simulink model "Solar_Farm_simulink"  (R2023a)
settings: Solver=FixedStepDiscrete  StartTime=0.0  StopTime=2.5  RelTol=1e-3
PreLoadFcn:
  | Ts_Power=1e-6;
  | Ts_Control=100e-6;
InitFcn:
  | Ts_Power=1e-6;
  | Ts_Control=100e-6;
undefined symbols (not defined in the file): D1, Delta, DiscIntNeverNeededParam
libraries: spsSeriesRLCBranchLib x5, spsMeanLib x3, spsThreePhaseTransformerTwoWindingsLib x2, spsDistributedParametersLineLib x2, spsThreePhaseParallelRLCLoadLib x2, spsFourierLib x2, slpidlib x2, spsabctodq0Lib x2, spsVoltageMeasurementLib x2, spsThreePhaseSeriesRLCLoadLib x1, spsThreeLevelBridgeLib x1, spsThreePhaseSourceLib x1
(part 1 of 2)
settings Model: SimulationMode=accelerator  Creator=The MathWorks, Inc.
settings SolverCC: AlgebraicLoopSolver=TrustRegion
settings DataIOCC: LimitDataPoints=on  SaveFormat=Array  SignalLogging=off  DSMLogging=off  ReturnWorkspaceOutputs=off
settings OptimizationCC: ExpressionDepthLimit=2147483647  EfficientMapNaN2IntZero=off  LifeSpan=inf
settings DebuggingCC: UnderspecifiedInitializationDetection=Classic  MergeDetectMultiDrivingBlocksExec=none  SolverPrmCheckMsg=warning  FcnCallInpInsideContextMsg=warning  UnconnectedInputMsg=warning  UnconnectedOutputMsg=warning  UnconnectedLineMsg=warning  StateNameClashWarn=warning  SFUnexpectedBacktrackingDiag=warning  SFNoUnconditionalDefaultTransitionDiag=warning  SFExecutionAtInitializationDiag=none  ArithmeticOperatorsInVariantConditions=warning
settings HardwareCC: ProdBitPerPointer=32  ProdBitPerSizeT=32  ProdBitPerPtrDiffT=32  ProdLargestAtomicFloat=None  ProdIntDivRoundTo=Undefined  ProdEndianess=Unspecified  ProdWordSize=32  ProdHWDeviceType=32-bit Generic  TargetBitPerLong=64  TargetBitPerPointer=64  TargetBitPerSizeT=64  TargetBitPerPtrDiffT=64  TargetLongLongMode=on  TargetIntDivRoundTo=Zero  TargetEndianess=LittleEndian  TargetWordSize=64  TargetHWDeviceType=MATLAB Host  ProdEqTarget=off
settings ModelReferenceCC: EnableRefExpFcnMdlSchedulingChecks=on  PropagateSignalLabelsOutOfModel=off
settings SFSimCC: SimUseLocalCustomCode=off  CustomCodeUndefinedFunction=UseInterfaceOnly
settings CodeAppCC: MaxIdLength=128
settings GRTTargetCC: TargetLangStandard=C89/C90 (ANSI)  CombineOutputUpdateFcns=off  GRTInterface=on
settings ConfigComp: CovMetricSettings=dw  CovSaveCumulativeToWorkspaceVar=on  CovSaveSingleToWorkspaceVar=on  CovExternalEMLEnable=off  CovSFcnEnable=off
settings SimscapeCC: SimscapeNormalizeSystem=off

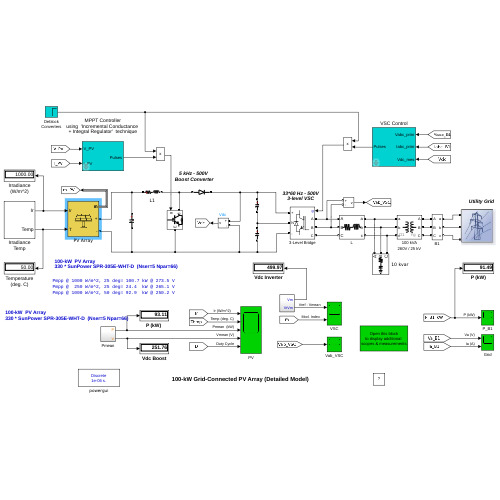
[thumbnail: Simulink's stored preview of the top-level diagram]
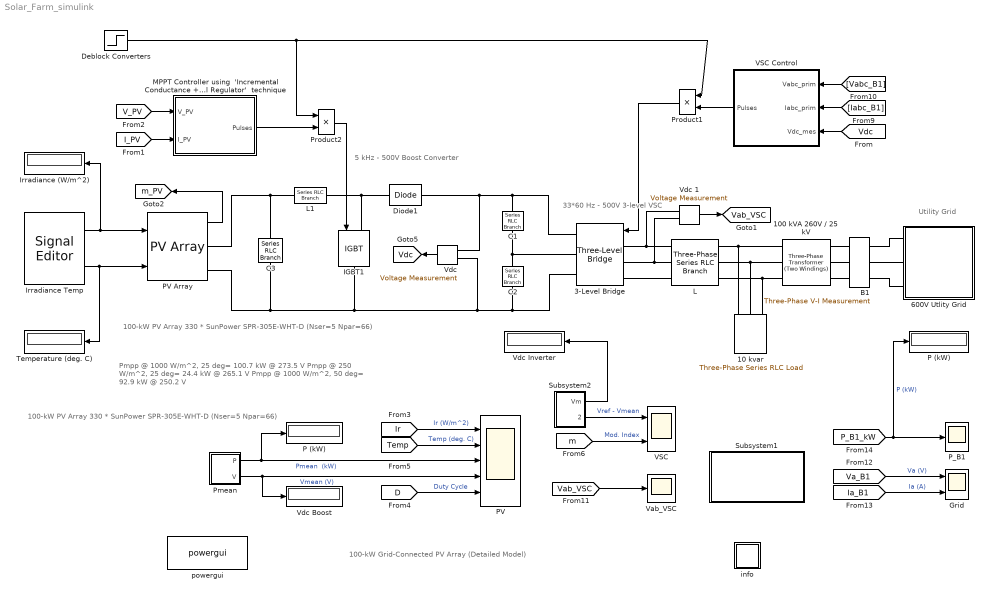
== system Solar_Farm_simulink ==
  note: 5 kHz - 500V
      | Boost Converter
  note: 33*60 Hz - 500V
      | 3-level VSC
  note: 100-kW Grid-Connected PV Array (Detailed Model)
  note: Utility Grid
  note: Pmpp @ 1000 W/m^2, 25 deg= 100.7 kW @ 273.5 V
      | Pmpp @  250 W/m^2, 25 deg= 24.4  kW @ 265.1 V
      | Pmpp @ 1000 W/m^2, 50 deg= 92.9  kW @ 250.2 V
  note: 100-kW  PV Array
      | 330 * SunPower SPR-305E-WHT-D  (Nser=5 Npar=66)
  note: 100-kW  PV Array
      | 330 * SunPower SPR-305E-WHT-D  (Nser=5 Npar=66)
  10 kvar : spsThreePhaseSeriesRLCLoadLib/Three-Phase Series RLC Load  LConnTagsString=A|B|C  Configuration=Y (grounded)  NominalVoltage=240  Vabc=[1e3 1e3 1e3]  Vabcp=[1e3 1e3 1e3]  NominalFrequency=60  UnbalancedPower=off  ActivePower=10e3/100  InductivePower=0  CapacitivePower=10e3  Pabc=[10e3 9e3 11e3]  QLabc=[100 90 110]  QCabc=[100 90 110]  Pabcp=[10e3 9e3 11e3]  QLabcp=[100 90 110]  QCabcp=[100 90 110]  Measurements=None  LoadType=constant Z
  100 kVA 260V / 25 kV : spsThreePhaseTransformerTwoWindingsLib/Three-Phase Transformer (Two Windings)  Winding1Connection=Yg  Winding2Connection=Delta (D1)  CoreType=Three single-phase transformers  SetSaturation=off  Hysteresis=off  DataFile='hysteresis'  SetInitialFlux=off  Measurements=None  UNITS=pu  NominalPower=[100e3 , 60 ]  Winding1=[ 25e3 , 0.001 , 0.03 ]  Winding2=[ 260 , 0.001 , 0.03 ]  Rm=500  Lm=500  L0=0.5  Saturation=[ 0,0 ; 0.0024,1.2 ; 1.0,1.52 ]  InitialFluxes=[ 0.8 , -0.8 , 0.7 ]  BreakLoop=off  DiscreteSolver=Trapezoidal iterative  DataType=off  TransfoNumber=0
  3-Level Bridge : spsThreeLevelBridgeLib/Three-Level Bridge  Arms=3  SnubberResistance=1e6  SbubberCapacitance=inf  Device=IGBT / Diodes  Ron=0.2e-3  ForwardVoltages="[  0  0 ]"  Measurements=None
      settings: AttributesFormatString=\n
  600V Utlity Grid : Subsystem
      mask Display: image('grid.jpg')
  B1 : spsThreePhaseVIMeasurementLib/Three-Phase V-I Measurement  VoltageMeasurement=phase-to-ground  SetLabelV=on  LabelV=Vabc_B1  Vpu=off  VpuLL=off  CurrentMeasurement=yes  SetLabelI=on  LabelI=Iabc_B1  Ipu=off  Pbase=100e6  Vbase=500e3  OutputType=Magnitude  PhasorSimulation=off  PSBequivalent=0
  C1 : spsSeriesRLCBranchLib/Series RLC Branch  LConnTagsString=__new0  RConnTagsString=__new0  BranchType=C  Resistance=1.0  Inductance=1.0  SetiL0=off  InitialCurrent=0  Capacitance=12000e-06  Setx0=off  InitialVoltage=0  Measurements=None
  C2 : spsSeriesRLCBranchLib/Series RLC Branch  LConnTagsString=__new0  RConnTagsString=__new0  BranchType=C  Resistance=1.0  Inductance=1.0  SetiL0=off  InitialCurrent=0  Capacitance=12000e-06  Setx0=off  InitialVoltage=0  Measurements=None
  C3 : spsSeriesRLCBranchLib/Series RLC Branch  LConnTagsString=__new0  RConnTagsString=__new0  BranchType=C  Resistance=1.0  Inductance=1.0  SetiL0=off  InitialCurrent=0  Capacitance=100e-6  Setx0=off  InitialVoltage=0  Measurements=Branch voltage
  Deblock Converters : Step  Time=0.05  SampleTime=0
  Diode1 : spsDiodeLib/Diode  Ron=1e-4  Lon=0  Vf=0  IC=0  UseSnubber=off  Rs=inf  Cs=inf  Measurements=off
  Grid : Scope  NumInputPorts=2
  IGBT1 : spsIGBTLib/IGBT  Ron=0.001  Lon=0  Vf=0  Tf=0  Tt=0  IC=0  Rs=1e5  Cs=inf  Measurements=off
  Irradiance (W/m^2) : Display
      settings: Format=bank  Decimation=1000
  Irradiance Temp : SignalEditorBlockLib/Signal Editor  FileName=dpower_PVarray_grid_det.mat  ActiveScenario=Ramp_up_down_Irradiance  ActiveSignal=Temp  IsBus=off  OutputBusObjectStr=Bus: BusObject  SampleTime=0  OutputAfterFinalValue=Extrapolation  Unit=inherit  PreserveSignalName=on  ApplySigPropsToAllScenarios=on
  L : spsThreePhaseSeriesRLCBranchLib/Three-Phase Series RLC Branch  LConnTagsString=A|B|C  RConnTagsString=A|B|C  BranchType=RL  Resistance=500e-6*377/50/2  Inductance=500e-6/2  Capacitance=inf  Measurements=None
  L1 : spsSeriesRLCBranchLib/Series RLC Branch  LConnTagsString=__new0  RConnTagsString=__new0  BranchType=RL  Resistance=0.005  Inductance=5e-3  SetiL0=off  InitialCurrent=0  Capacitance=1e-6  Setx0=off  InitialVoltage=0  Measurements=None
  "MPPT Controller using  'Incremental Conductance + Integral Regulator'  technique " : Subsystem  mask(Boost Control - MPPT){fc=5000, T_MPPT=200e-6, Dinit=0.5}
      mask prompts: fc "PWM switching frequency (Hz)"; T_MPPT "Time window used by MPPT control (s)"; Dinit "Initial value of duty cycle"
  P (kW) : Display
      settings: Format=bank  Decimation=2000
  "P (kW) " : Display
      settings: Format=bank  Decimation=2000
  PV : Scope  NumInputPorts=5
  PV Array : spsPVArrayLib/PV Array  Npar=66  Nser=5  PlotType=array @ 1000 W/m2 & specified temperatures  S_vec="[ 1000  250 ]"  Temp_C_vec="[0 25  50  ]"  ModuleName=SunPower SPR-305E-WHT-D  PlotWhenSelected=off  Pm=305.226  Ncell=96  Voc=64.2  Isc=5.96  Vm=54.7  Im=5.58  beta_Voc_pc=-0.2727  alpha_Isc_pc=0.061745  beta_Voc=-0.17507  alpha_Isc=0.00368  IL=5.9657  I0=6.3076e-12  nI=0.94489  Rsh=393.2054  Rs=0.37428  RobustModel=off  RobustCellTemperature=25  BAL=on  Tc=1e-6  Tfilter=5e-5
  P_B1 : Scope
  Pmean : Subsystem
  Product1 : Product  RndMeth=Zero
  Product2 : Product  RndMeth=Zero
  Subsystem1 : Subsystem
      mask Display: disp('Open this block\nto display additional \nscopes & measurements')
  Subsystem2 : Subsystem
  Temperature (deg. C) : Display
      settings: Format=bank  Decimation=1000
  VSC : Scope  NumInputPorts=2
  VSC Control : Subsystem  mask(VSC Main Controller){nom=[ 100e3  60 ], Vnom=[ 25e3 260 ], Vnom_dc=500, RLxfo=[0.002  0.06 ], RLchoke=[2e-3  250e-6  ], K_VDCreg=[7  800], K_Ireg=[0.3 20], Ts=Ts_Control}
      mask prompts: nom "Nominal power and frequency [ Pnom(VA)  Fnom(Hz) ]:"; Vnom "Nominal primary and secondary voltages (Vrms LL) [ Vnom_prim   Vnom_sec ]:"; Vnom_dc "Nominal DC bus voltage (V):"; RLxfo "Total transformer leakage impedance (pu/Pnom) [ Rxfo  Lxf ]"; RLchoke "Choke impedance [ R(ohm) L(H) ]"; K_VDCreg "VDC regultator gains [ Kp  Ki ]:"; K_Ireg "Current regulator gains [ Kp  Ki ]:"; Ts "Sample time"
      mask init:
      | Pnom=nom(1);
      | Fnom=nom(2);
      | Vnom_prim=Vnom(1);
      | Vnom_sec=Vnom(2);
      | Zbase=Vnom_sec^2/Pnom;
      | Rtot_pu=RLxfo(1) + RLchoke(1)/Zbase;
      | Ltot_pu=RLxfo(2) + RLchoke(2)/(Zbase/(2*pi*Fnom));
      | Kp_VDCreg=K_VDCreg(1);
      | Ki_VDCreg=K_VDCreg(2);
      | Kp_Ireg=K_Ireg(1);
      | Ki_Ireg=K_Ireg(2);
      | Vdc_ref=Vnom_dc;
      | % Used to determine initial value of Boost Control (MPPT)
      | assignin('base','Vdc_ref_Inv',Vdc_ref);
  Vab_VSC : Scope
  "Vdc " : spsVoltageMeasurementLib/Voltage Measurement  Tag=PoWeRsYsTeMmEaSuReMeNt  PhasorSimulation=off  OutputType=Magnitude  PSBequivalent=0
  Vdc 1 : spsVoltageMeasurementLib/Voltage Measurement  Tag=PoWeRsYsTeMmEaSuReMeNt  PhasorSimulation=off  OutputType=Magnitude  PSBequivalent=0
  Vdc Boost : Display
      settings: Format=bank  Decimation=2000
  Vdc Inverter : Display
      settings: Format=bank  Decimation=2000
  info : Subsystem
      settings: OpenFcn=showdemo(bdroot(gcb))
      mask Display: disp('?')
  powergui : spspowerguiLib/powergui  Priority=1  SimulationMode=Discrete  SampleTime=Ts_Power  frequency=60  Iterations=50  frequencyindice=0  Pbase=100e6  ErrMax=1e-4  UnitsV=kV  UnitsW=MW  buscounter=0  FunctionMessages=off  echomessages=off  EnableUseOfTLC=off  CurrentSourceSwitches=off  DisableSnubberDevices=off  DisableRonSwitches=off  DisableVfSwitches=off  DisplayEquations=off  AutomaticDiscreteSolvers=off  SolverType=Tustin/Backward Euler (TBE)  Interpol=off  ExternalGateDelay=off  methode=off  Ts=0  x0status=blocks  SPID=off  SwTol=0  HookPort=off  NonlinearTolerance=1e-8  nMaxIteration=10  ContinueOnMaxIteration=off  RestoreLinks=warning  ResistiveCurrentMeasurement=off  Frange=[0:2:500]  Ylog=off  Xlog=on  ShowGrid=off  save=off  variable=ZData  structure=0  ZoomFFT=on  StartTime=0.0  cycles=1  DisplayStyle=1  fundamental=60  FreqAxis=off  MaxFrequency=1000  frequencyindicesteady=1  RmsSteady=1  display=off
  tag scope: Vab_VSC=global, Vdc=global, m_PV=global
  wires:
  "Vdc "/1 -> [Vdc]
  Product2/1 -> IGBT1/1
  "MPPT Controller using  'Incremental Conductance + Integral Regulator'  technique "/1(Pulses) -> Product2/2
  Deblock Converters/1 -> Product1/1, Product2/1
  [Vabc_B1] -> VSC Control/1(Vabc_prim)
  [Iabc_B1] -> VSC Control/2(Iabc_prim)
  [Vdc] -> VSC Control/3(Vdc_mes)
  VSC Control/1(Pulses) -> Product1/2
  Product1/1 -> 3-Level Bridge/1
  [I_PV] -> "MPPT Controller using  'Incremental Conductance + Integral Regulator'  technique "/2(I_PV)
  [V_PV] -> "MPPT Controller using  'Incremental Conductance + Integral Regulator'  technique "/1(V_PV)
  Pmean/1(P) -> "P (kW) "/1, PV/3  "Pmean  (kW)"
  [m] -> VSC/2  "Mod. Index"
  Vdc 1/1 -> [Vab_VSC]
  [Vab_VSC] -> Vab_VSC/1
  [Ia_B1] -> Grid/2  "Ia (A)"
  [Va_B1] -> Grid/1  "Va (V)"
  [P_B1_kW] -> P_B1/1, P (kW)/1  "P (kW)"
  Pmean/2(V) -> Vdc Boost/1, PV/4  "Vmean (V)"
  Subsystem2/2(VrVm) -> VSC/1  "Vref - Vmean"
  Subsystem2/1(Vm) -> Vdc Inverter/1
  PV Array/1 -> [m_PV]
  Irradiance Temp/1 -> PV Array/1, Irradiance (W/m^2)/1
  Irradiance Temp/2 -> PV Array/2, Temperature (deg. C)/1
  [D] -> PV/5  "Duty Cycle"
  [Temp] -> PV/2  "Temp (deg. C)"
  [Ir] -> PV/1  "Ir (W/m^2)"
  connections:
  3-Level Bridge/RConn1 -- Diode1/RConn1 -- "Vdc "/LConn1 -- C1/LConn1
  L1/RConn1 -- Diode1/LConn1 -- IGBT1/LConn1
  3-Level Bridge/RConn3 -- C2/RConn1 -- "Vdc "/LConn2 -- IGBT1/RConn1 -- PV Array/RConn2 -- C3/RConn1
  3-Level Bridge/LConn1 -- L/LConn1 -- Vdc 1/LConn1
  3-Level Bridge/LConn2 -- L/LConn2 -- Vdc 1/LConn2
  3-Level Bridge/LConn3 -- L/LConn3
  L/RConn1 -- 100 kVA 260V / 25 kV/RConn1 -- 10 kvar/LConn1
  L/RConn2 -- 100 kVA 260V / 25 kV/RConn2 -- 10 kvar/LConn2
  L/RConn3 -- 100 kVA 260V / 25 kV/RConn3 -- 10 kvar/LConn3
  B1/LConn1 -- 100 kVA 260V / 25 kV/LConn1
  B1/LConn2 -- 100 kVA 260V / 25 kV/LConn2
  B1/LConn3 -- 100 kVA 260V / 25 kV/LConn3
  C2/LConn1 -- C1/RConn1 -- 3-Level Bridge/RConn2
  C3/LConn1 -- PV Array/RConn1 -- L1/LConn1
  B1/RConn2 -- 600V Utlity Grid/LConn2
  B1/RConn1 -- 600V Utlity Grid/LConn1
  B1/RConn3 -- 600V Utlity Grid/LConn3

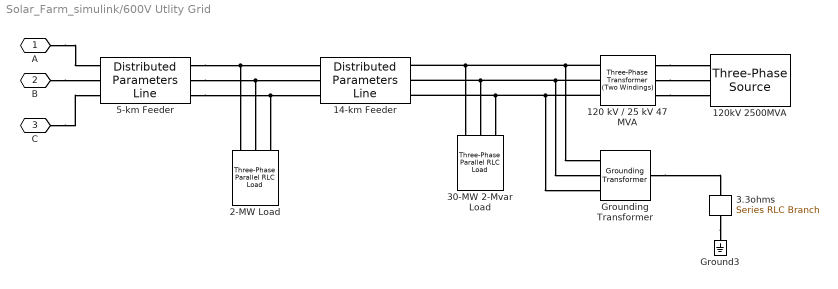
== system Solar_Farm_simulink/600V Utlity Grid ==
  120 kV / 25 kV 47 MVA : spsThreePhaseTransformerTwoWindingsLib/Three-Phase Transformer (Two Windings)  Winding1Connection=Yg  Winding2Connection=Delta (D1)  CoreType=Three single-phase transformers  SetSaturation=off  Hysteresis=off  DataFile='basic_model'  SetInitialFlux=off  Measurements=None  UNITS=pu  NominalPower=[47e6 60 ]  Winding1="[ 120e3  0.08/30   0.08 ]"  Winding2="[ 25e3  0.08/30  0.08]"  Rm=500  Lm=500  L0=0.5  Saturation="[ 0,0  ;  0.005,1.2  ;  1.0,1.4 ]"  InitialFluxes=[ 0.8 , -0.8 , 0.7 ]  BreakLoop=off  DiscreteSolver=Trapezoidal iterative  DataType=off  TransfoNumber=0
  120kV 2500MVA : spsThreePhaseSourceLib/Three-Phase Source  InternalConnection=Yg  VoltagePhases=off  Voltage=120e3  PhaseAngle=0  Voltage_phases=[25e3 25e3 25e3]/sqrt(3)  PhaseAngles_phases=[0 -120 +120]  Frequency=60  NonIdealSource=on  SpecifyImpedance=on  Resistance=0.8929  Inductance=16.58e-3  ShortCircuitLevel=2500e6  BaseVoltage=120e3  XRratio=7  BusType=swing  Pref=0  Qref=0  Prefabc=[10e3, 10e3, 10e3]  Qrefabc=[0, 0, 0]  Qmin=-inf  Qmax=inf
  14-km Feeder : spsDistributedParametersLineLib/Distributed Parameters Line  Phases=3  Length=14  Frequency=60  Resistance=[0.1153 0.413]  Inductance=[1.05e-3 3.32e-3]  Capacitance=[11.33e-009 5.01e-009]  x1=[-5.8e-05 2.50217396067509e-09 0 0;-5.7e-05 2.50196188940633e-09 0 0;-5.6e-05 2.50174946255299e-09 0 0;-5.5e-05 2.50153668014525e-09 0 0;-5.4e-05 2.50132354221337e-09 0 0;-5.3e-05 2.50111004878763e-09 0 0;-5.2e-05 2.50089619989837e-09 0 0;-5.1e-05 2.50068199557598e-09 0 0;-5e-05 2.50046743585092e-09 0 0;-4.9e-05 2.50025252075366e-09 -3790.73535189975 -24061.4134200279;-4.8e-05 2.50003725031477e-09 -3781.66414358436 -24062.8407837223;-4.7e-05 2.49982162456482e-09 -3772.59239781015 -24064.2647275504;-4.6e-05 2.49960564353448e-09 -3763.52011586643 -24065.6852513098;-4.5e-05 2.49938930725442e-09 -3754.44729904257 -24067.1023547986;-4.4e-05 2.49917261575541e-09 -3745.37394862801 -24068.5160378155;-4.3e-05 2.49895556906823e-09 -3736.30006591229 -24069.9263001594;-4.2e-05 2.49873816722373e-09 -3727.225652185 -24071.33314163;-4.1e-05 2.49852041025281e-09 -3718.15070873583 -24072.7365620274;-4e-05 2.49830229818642e-09 -3709.07523685452 -24074.136561152;-3.9e-05 2.49808383105556e-09 -3699.99923783089 -24075.5331388049;-3.8e-05 2.49786500889127e-09 -3690.92271295487 -24076.9262947876;-3.7e-05 2.49764583172466e-09 -3681.8456635164 -24078.3160289022;-3.6e-05 2.49742629958688e-09 -3672.76809080556 -24079.702340951;-3.5e-05 2.49720641250912e-09 -3663.68999611247 -24081.0852307371;-3.4e-05 2.49698617052264e-09 -3654.61138072732 -24082.464698064;-3.3e-05 2.49676557365874e-09 -3645.53224594039 -24083.8407427356;-3.2e-05 2.49654462194876e-09 -3636.45259304202 -24085.2133645562;-3.1e-05 2.49632331542412e-09 -3627.37242332264 -24086.582563331;-3e-05 2.49610165411627e-09 -3618.29173807275 -24087.9483388651;-2.9e-05 2.4958796380567e-09 -3609.2105385829 -24089.3106909646;-2.8e-05 2.49565726727697e-09 -3600.12882614375 -24090.6696194359;-2.7e-05 2.49543454180869e-09 -3591.046602046 -24092.0251240857;-2.6e-05 2.4952114616835e-09 -3581.96386758044 -24093.3772047214;-2.5e-05 2.49498802693312e-09 -3572.88062403793 -24094.7258611509;-2.4e-05 2.4947642375893e-09 -3563.7968727094 -24096.0710931825;-2.3e-05 2.49454009368384e-09 -3554.71261488586 -24097.4129006251;-2.2e-05 2.49431559524861e-09 -3545.62785185838 -24098.7512832878;-2.1e-05 2.4940907423155e-09 -3536.54258491811 -24100.0862409806;-2e-05 2.49386553491647e-09 -3527.45681535627 -24101.4177735136;-1.9e-05 2.49363997308353e-09 -3518.37054446415 -24102.7458806977;-1.8e-05 2.49341405684874e-09 -3509.2837735331 -24104.070562344;-1.7e-05 2.49318778624421e-09 -3500.19650385457 -24105.3918182643;-1.6e-05 2.49296116130209e-09 -3491.10873672006 -24106.7096482709;-1.5e-05 2.49273418205459e-09 -3482.02047342113 -24108.0240521764;-1.4e-05 2.49250684853397e-09 -3472.93171524945 -24109.3350297941;-1.3e-05 2.49227916077254e-09 -3463.84246349671 -24110.6425809375;-1.2e-05 2.49205111880266e-09 -3454.75271945471 -24111.946705421;-1.1e-05 2.49182272265674e-09 -3445.6624844153 -24113.247403059;-1e-05 2.49159397236724e-09 -3436.57175967041 -24114.5446736669;-9e-06 2.49136486796667e-09 -3427.48054651203 -24115.8385170602;-8e-06 2.49113540948759e-09 -3418.38884623222 -24117.1289330549;-7e-06 2.49090559696261e-09 -3409.29666012313 -24118.4159214678;-6e-06 2.49067543042439e-09 -3400.20398947694 -24119.699482116;-5e-06 2.49044490990565e-09 -3391.11083558594 -24120.9796148169;-4e-06 2.49021403543915e-09 -3382.01719974246 -24122.2563193887;-3e-06 2.48998280705769e-09 -3372.92308323891 -24123.5295956499;-2e-06 2.48975122479415e-09 -3363.82848736777 -24124.7994434195;-1e-06 2.48951928868143e-09 -3354.73341342159 -24126.0658625171]  x2=[-5.8e-05 2.62043607139288e-09 0 0;-5.7e-05 2.62017695324581e-09 0 0;-5.6e-05 2.61991746271315e-09 0 0;-5.5e-05 2.61965759983179e-09 0 0;-5.4e-05 2.61939736463867e-09 0 0;-5.3e-05 2.61913675717076e-09 0 0;-5.2e-05 2.61887577746511e-09 0 0;-5.1e-05 2.6186144255588e-09 0 0;-5e-05 2.61835270148898e-09 0 0;-4.9e-05 2.61809060529286e-09 -3379.39242591326 -24244.0512732181;-4.8e-05 2.61782813700767e-09 -3370.25239398146 -24245.323551308;-4.7e-05 2.61756529667072e-09 -3361.11188306163 -24246.5923835967;-4.6e-05 2.61730208431936e-09 -3351.97089445284 -24247.8577699039;-4.5e-05 2.61703849999101e-09 -3342.82942945423 -24249.1197100497;-4.4e-05 2.61677454372312e-09 -3333.68748936501 -24250.3782038548;-4.3e-05 2.61651021555321e-09 -3324.54507548445 -24251.6332511404;-4.2e-05 2.61624551551885e-09 -3315.4021891119 -24252.884851728;-4.1e-05 2.61598044365765e-09 -3306.25883154675 -24254.1330054398;-4e-05 2.61571500000729e-09 -3297.11500408849 -24255.3777120984;-3.9e-05 2.6154491846055e-09 -3287.97070803665 -24256.6189715269;-3.8e-05 2.61518299749005e-09 -3278.82594469085 -24257.8567835489;-3.7e-05 2.61491643869877e-09 -3269.68071535076 -24259.0911479884;-3.6e-05 2.61464950826954e-09 -3260.53502131612 -24260.3220646701;-3.5e-05 2.61438220624031e-09 -3251.38886388674 -24261.5495334189;-3.4e-05 2.61411453264907e-09 -3242.24224436249 -24262.7735540605;-3.3e-05 2.61384648753385e-09 -3233.09516404331 -24263.9941264209;-3.2e-05 2.61357807093275e-09 -3223.9476242292 -24265.2112503265;-3.1e-05 2.61330928288392e-09 -3214.79962622023 -24266.4249256045;-3e-05 2.61304012342556e-09 -3205.65117131655 -24267.6351520823;-2.9e-05 2.61277059259592e-09 -3196.50226081834 -24268.841929588;-2.8e-05 2.61250069043331e-09 -3187.35289602587 -24270.04525795;-2.7e-05 2.61223041697609e-09 -3178.20307823947 -24271.2451369973;-2.6e-05 2.61195977226267e-09 -3169.05280875954 -24272.4415665594;-2.5e-05 2.61168875633152e-09 -3159.90208888652 -24273.6345464662;-2.4e-05 2.61141736922115e-09 -3150.75091992095 -24274.8240765482;-2.3e-05 2.61114561097013e-09 -3141.5993031634 -24276.0101566363;-2.2e-05 2.61087348161709e-09 -3132.44723991454 -24277.192786562;-2.1e-05 2.6106009812007e-09 -3123.29473147505 -24278.3719661572;-2e-05 2.61032810975968e-09 -3114.14177914574 -24279.5476952542;-1.9e-05 2.61005486733283e-09 -3104.98838422742 -24280.7199736861;-1.8e-05 2.60978125395898e-09 -3095.83454802101 -24281.8888012861;-1.7e-05 2.609507269677e-09 -3086.68027182747 -24283.0541778883;-1.6e-05 2.60923291452585e-09 -3077.52555694782 -24284.2161033268;-1.5e-05 2.60895818854451e-09 -3068.37040468316 -24285.3745774367;-1.4e-05 2.60868309177202e-09 -3059.21481633464 -24286.5296000533;-1.3e-05 2.60840762424749e-09 -3050.05879320346 -24287.6811710123;-1.2e-05 2.60813178601007e-09 -3040.9023365909 -24288.8292901503;-1.1e-05 2.60785557709895e-09 -3031.74544779831 -24289.9739573039;-1e-05 2.6075789975534e-09 -3022.58812812708 -24291.1151723104;-9e-06 2.60730204741271e-09 -3013.43037887866 -24292.2529350078;-8e-06 2.60702472671626e-09 -3004.27220135458 -24293.3872452343;-7e-06 2.60674703550346e-09 -2995.11359685643 -24294.5181028287;-6e-06 2.60646897381376e-09 -2985.95456668583 -24295.6455076302;-5e-06 2.6061905416867e-09 -2976.7951121445 -24296.7694594787;-4e-06 2.60591173916183e-09 -2967.63523453419 -24297.8899582144;-3e-06 2.6056325662788e-09 -2958.47493515674 -24299.007003678;-2e-06 2.60535302307726e-09 -2949.31421531402 -24300.1205957109;-1e-06 2.60507310959696e-09 -2940.15307630797 -24301.2307341546]  x3=[-5.8e-05 1.12841261134887e-11 0 0;-5.7e-05 1.12856673900563e-11 0 0;-5.6e-05 1.12872070626789e-11 0 0;-5.5e-05 1.12887451311376e-11 0 0;-5.4e-05 1.12902815952139e-11 0 0;-5.3e-05 1.12918164546894e-11 0 0;-5.2e-05 1.1293349709346e-11 0 0;-5.1e-05 1.12948813589657e-11 0 0;-5e-05 1.12964114033308e-11 0 0;-4.9e-05 1.1297939842224e-11 -23.5442847382639 -155.681477773843;-4.8e-05 1.1299466675428e-11 -23.4855925321452 -155.690342696964;-4.7e-05 1.13009919027257e-11 -23.4268969882001 -155.699185493015;-4.6e-05 1.13025155239005e-11 -23.3681981147704 -155.70800616074;-4.5e-05 1.13040375387357e-11 -23.3094959201986 -155.716804698884;-4.4e-05 1.13055579470151e-11 -23.2507904128276 -155.725581106197;-4.3e-05 1.13070767485226e-11 -23.1920816010008 -155.734335381433;-4.2e-05 1.13085939430424e-11 -23.133369493062 -155.743067523346;-4.1e-05 1.13101095303587e-11 -23.0746540973554 -155.751777530696;-4e-05 1.13116235102562e-11 -23.0159354222259 -155.760465402245;-3.9e-05 1.13131358825198e-11 -22.9572134760186 -155.769131136758;-3.8e-05 1.13146466469344e-11 -22.8984882670794 -155.777774733004;-3.7e-05 1.13161558032854e-11 -22.8397598037543 -155.786396189754;-3.6e-05 1.13176633513583e-11 -22.7810280943899 -155.794995505782;-3.5e-05 1.13191692909389e-11 -22.7222931473334 -155.803572679867;-3.4e-05 1.1320673621813e-11 -22.6635549709323 -155.81212771079;-3.3e-05 1.1322176343767e-11 -22.6048135735346 -155.820660597335;-3.2e-05 1.13236774565872e-11 -22.5460689634888 -155.829171338288;-3.1e-05 1.13251769600603e-11 -22.4873211491437 -155.837659932442;-3e-05 1.13266748539732e-11 -22.4285701388489 -155.846126378588;-2.9e-05 1.13281711381129e-11 -22.369815940954 -155.854570675524;-2.8e-05 1.1329665812267e-11 -22.3110585638093 -155.86299282205;-2.7e-05 1.13311588762228e-11 -22.2522980157657 -155.871392816968;-2.6e-05 1.13326503297683e-11 -22.1935343051743 -155.879770659086;-2.5e-05 1.13341401726914e-11 -22.1347674403867 -155.888126347211;-2.4e-05 1.13356284047804e-11 -22.0759974297549 -155.896459880157;-2.3e-05 1.13371150258238e-11 -22.0172242816317 -155.90477125674;-2.2e-05 1.13386000356103e-11 -21.9584480043698 -155.913060475777;-2.1e-05 1.13400834339289e-11 -21.8996686063228 -155.921327536092;-2e-05 1.13415652205688e-11 -21.8408860958444 -155.929572436509;-1.9e-05 1.13430453953193e-11 -21.7821004812891 -155.937795175856;-1.8e-05 1.13445239579701e-11 -21.7233117710114 -155.945995752964;-1.7e-05 1.1346000908311e-11 -21.6645199733668 -155.954174166669;-1.6e-05 1.13474762461321e-11 -21.6057250967106 -155.962330415807;-1.5e-05 1.13489499712238e-11 -21.5469271493991 -155.97046449922;-1.4e-05 1.13504220833766e-11 -21.4881261397888 -155.978576415752;-1.3e-05 1.13518925823813e-11 -21.4293220762364 -155.986666164249;-1.2e-05 1.13533614680289e-11 -21.3705149670995 -155.994733743563;-1.1e-05 1.13548287401107e-11 -21.3117048207358 -156.002779152545;-1e-05 1.1356294398418e-11 -21.2528916455036 -156.010802390054;-9e-06 1.13577584427427e-11 -21.1940754497615 -156.018803454949;-8e-06 1.13592208728765e-11 -21.1352562418686 -156.026782346091;-7e-06 1.13606816886118e-11 -21.0764340301845 -156.034739062349;-6e-06 1.13621408897408e-11 -21.017608823069 -156.04267360259;-5e-06 1.13635984760562e-11 -20.9587806288826 -156.050585965687;-4e-06 1.13650544473509e-11 -20.8999494559861 -156.058476150516;-3e-06 1.13665088034178e-11 -20.8411153127406 -156.066344155955;-2e-06 1.13679615440503e-11 -20.7822782075078 -156.074189980886;-1e-06 1.1369412669042e-11 -20.7234381486499 -156.082013624194]  x4=[-5.8e-05 -5.62786037485921e-12 0 0;-5.7e-05 -5.62923828223865e-12 0 0;-5.6e-05 -5.63061538957779e-12 0 0;-5.5e-05 -5.63199169668091e-12 0 0;-5.4e-05 -5.6333672033524e-12 0 0;-5.3e-05 -5.63474190939679e-12 0 0;-5.2e-05 -5.63611581461868e-12 0 0;-5.1e-05 -5.63748891882282e-12 0 0;-5e-05 -5.63886122181406e-12 0 0;-4.9e-05 -5.64023272339737e-12 -1.35581366009314 -2.15298522698133;-4.8e-05 -5.64160342337782e-12 -1.355001907458 -2.15349620368372;-4.7e-05 -5.6429733215606e-12 -1.35418996224687 -2.15400687432627;-4.6e-05 -5.64434241775103e-12 -1.35337782457515 -2.1545172388364;-4.5e-05 -5.64571071175452e-12 -1.35256549455825 -2.15502729714159;-4.4e-05 -5.64707820337661e-12 -1.35175297231164 -2.15553704916934;-4.3e-05 -5.64844489242295e-12 -1.35094025795078 -2.1560464948472;-4.2e-05 -5.6498107786993e-12 -1.35012735159118 -2.15655563410277;-4.1e-05 -5.65117586201154e-12 -1.34931425334838 -2.15706446686369;-4e-05 -5.65254014216565e-12 -1.34850096333792 -2.15757299305764;-3.9e-05 -5.65390361896775e-12 -1.34768748167541 -2.15808121261235;-3.8e-05 -5.65526629222406e-12 -1.34687380847645 -2.15858912545559;-3.7e-05 -5.6566281617409e-12 -1.34605994385669 -2.15909673151518;-3.6e-05 -5.65798922732473e-12 -1.34524588793178 -2.15960403071897;-3.5e-05 -5.65934948878211e-12 -1.34443164081744 -2.16011102299487;-3.4e-05 -5.66070894591971e-12 -1.34361720262937 -2.16061770827082;-3.3e-05 -5.66206759854433e-12 -1.34280257348334 -2.1611240864748;-3.2e-05 -5.66342544646287e-12 -1.34198775349511 -2.16163015753485;-3.1e-05 -5.66478248948234e-12 -1.3411727427805 -2.16213592137905;-3e-05 -5.6661387274099e-12 -1.34035754145533 -2.16264137793552;-2.9e-05 -5.66749416005277e-12 -1.33954214963546 -2.16314652713242;-2.8e-05 -5.66884878721833e-12 -1.33872656743677 -2.16365136889795;-2.7e-05 -5.67020260871405e-12 -1.33791079497519 -2.16415590316037;-2.6e-05 -5.67155562434753e-12 -1.33709483236664 -2.16466012984798;-2.5e-05 -5.67290783392646e-12 -1.3362786797271 -2.1651640488891;-2.4e-05 -5.67425923725868e-12 -1.33546233717256 -2.16566766021212;-2.3e-05 -5.67560983415212e-12 -1.33464580481903 -2.16617096374548;-2.2e-05 -5.67695962441482e-12 -1.33382908278257 -2.16667395941762;-2.1e-05 -5.67830860785495e-12 -1.33301217117925 -2.16717664715708;-2e-05 -5.67965678428079e-12 -1.33219507012518 -2.16767902689241;-1.9e-05 -5.68100415350074e-12 -1.33137777973647 -2.1681810985522;-1.8e-05 -5.68235071532331e-12 -1.33056030012929 -2.1686828620651;-1.7e-05 -5.6836964695571e-12 -1.32974263141982 -2.16918431735981;-1.6e-05 -5.68504141601088e-12 -1.32892477372426 -2.16968546436505;-1.5e-05 -5.68638555449348e-12 -1.32810672715886 -2.17018630300959;-1.4e-05 -5.68772888481389e-12 -1.32728849183987 -2.17068683322226;-1.3e-05 -5.68907140678117e-12 -1.32647006788359 -2.17118705493192;-1.2e-05 -5.69041312020452e-12 -1.32565145540633 -2.17168696806749;-1.1e-05 -5.69175402489327e-12 -1.32483265452443 -2.1721865725579;-1e-05 -5.69309412065684e-12 -1.32401366535426 -2.17268586833215;-9e-06 -5.69443340730476e-12 -1.32319448801223 -2.17318485531929;-8e-06 -5.6957718846467e-12 -1.32237512261475 -2.1736835334484;-7e-06 -5.69710955249243e-12 -1.32155556927827 -2.17418190264859;-6e-06 -5.69844641065184e-12 -1.32073582811927 -2.17467996284906;-5e-06 -5.69978245893493e-12 -1.31991589925426 -2.175177713979;-4e-06 -5.70111769715182e-12 -1.31909578279976 -2.17567515596767;-3e-06 -5.70245212511274e-12 -1.31827547887233 -2.17617228874439;-2e-06 -5.70378574262803e-12 -1.31745498758856 -2.17666911223849;-1e-06 -5.70511854950817e-12 -1.31663430906506 -2.17716562637937]  x5=5.70973484498186e-05  V1=[0 0 0 2.868e-09 2.436e+04 2.436e+04;0 0 0 377 377 377;1.571 1.571 1.571 -0.5389 -0.156 -1.727]  V2=[0 0 0 2.996e-09 2.448e+04 2.448e+04;0 0 0 377 377 377;1.571 1.571 1.571 -0.5232 -0.1382 -1.709]  I1=[0 0 0 1.022e-11 157.5 157.5;0 0 0 377 377 377;1.571 1.571 1.571 -1.198 -0.1498 -1.721]  I2=[0 0 0 6.231e-12 2.544 2.544;0 0 0 377 377 377;1.571 1.571 1.571 1.184 -0.5617 -2.133]  nHarmo=2  Measurements=None  Decoupling=off  VsMag0=0  VrMag0=0  VsAngle0=0  VrAngle0=0  IsMag0=0  IrMag0=0  IsAngle0=0  IrAngle0=0
  2-MW Load : spsThreePhaseParallelRLCLoadLib/Three-Phase Parallel RLC Load  LConnTagsString=A|B|C  Configuration=Y (grounded)  NominalVoltage=25e3  Vabc=[1e3 1e3 1e3]  Vabcp=[1e3 1e3 1e3]  NominalFrequency=60  UnbalancedPower=off  ActivePower=2e6  InductivePower=0  CapacitivePower=0  Pabc=[10e3 9e3 11e3]  QLabc=[100 90 110]  QCabc=[100 90 110]  Pabcp=[10e3 9e3 11e3]  QLabcp=[100 90 110]  QCabcp=[100 90 110]  Measurements=None  LoadType=constant Z
  "3.3ohms " : spsSeriesRLCBranchLib/Series RLC Branch  LConnTagsString=__new0  RConnTagsString=__new0  BranchType=R  Resistance=3.3  Inductance=[]  SetiL0=off  InitialCurrent=0  Capacitance=[]  Setx0=off  InitialVoltage=0  Measurements=None
  30-MW 2-Mvar Load : spsThreePhaseParallelRLCLoadLib/Three-Phase Parallel RLC Load  LConnTagsString=A|B|C  Configuration=Y (grounded)  NominalVoltage=25e3  Vabc=[1e3 1e3 1e3]  Vabcp=[1e3 1e3 1e3]  NominalFrequency=60  UnbalancedPower=off  ActivePower=30e6  InductivePower=2e6  CapacitivePower=0  Pabc=[10e3 9e3 11e3]  QLabc=[100 90 110]  QCabc=[100 90 110]  Pabcp=[10e3 9e3 11e3]  QLabcp=[100 90 110]  QCabcp=[100 90 110]  Measurements=None  LoadType=constant Z
  5-km Feeder : spsDistributedParametersLineLib/Distributed Parameters Line  Phases=3  Length=5  Frequency=60  Resistance=[0.1153 0.413]  Inductance=[1.05e-3 3.32e-3]  Capacitance=[11.33e-009 5.01e-009]  x1=[-2.1e-05 2.44326143824986e-09 -3537.17773129636 -24101.4118174718;-2e-05 2.44303128240586e-09 -3528.09146195883 -24102.7435893552;-1.9e-05 2.44280077935263e-09 -3519.00469120083 -24104.0719357012;-1.8e-05 2.44256992912293e-09 -3509.91742031377 -24105.396856321;-1.7e-05 2.44233873174956e-09 -3500.82965058918 -24106.7183510263;-1.6e-05 2.4421071872654e-09 -3491.74138331861 -24108.0364196293;-1.5e-05 2.44187529570334e-09 -3482.65261979372 -24109.3510619426;-1.4e-05 2.44164305709634e-09 -3473.56336130623 -24110.6622777795;-1.3e-05 2.44141047147742e-09 -3464.47360914792 -24111.9700669536;-1.2e-05 2.44117753887961e-09 -3455.38336461064 -24113.274429279;-1.1e-05 2.44094425933604e-09 -3446.29262898633 -24114.5753645704;-1e-05 2.44071063287985e-09 -3437.20140356697 -24115.8728726428;-9e-06 2.44047665954425e-09 -3428.10968964464 -24117.1669533118;-8e-06 2.44024233936248e-09 -3419.01748851147 -24118.4576063935;-7e-06 2.44000767236786e-09 -3409.92480145967 -24119.7448317046;-6e-06 2.43977265859374e-09 -3400.8316297815 -24121.028629062;-5e-06 2.4395372980735e-09 -3391.73797476932 -24122.3089982833;-4e-06 2.43930159084061e-09 -3382.64383771553 -24123.5859391865;-3e-06 2.43906553692857e-09 -3373.54921991261 -24124.8594515901;-2e-06 2.43882913637091e-09 -3364.45412265311 -24126.1295353132;-1e-06 2.43859238920125e-09 -3355.35854722965 -24127.3961901752]  x2=[-2.1e-05 2.4940907423155e-09 -3536.54258491811 -24100.0862409806;-2e-05 2.49386553491647e-09 -3527.45681535627 -24101.4177735136;-1.9e-05 2.49363997308353e-09 -3518.37054446415 -24102.7458806977;-1.8e-05 2.49341405684874e-09 -3509.2837735331 -24104.070562344;-1.7e-05 2.49318778624421e-09 -3500.19650385457 -24105.3918182643;-1.6e-05 2.49296116130209e-09 -3491.10873672006 -24106.7096482709;-1.5e-05 2.49273418205459e-09 -3482.02047342113 -24108.0240521764;-1.4e-05 2.49250684853397e-09 -3472.93171524945 -24109.3350297941;-1.3e-05 2.49227916077254e-09 -3463.84246349671 -24110.6425809375;-1.2e-05 2.49205111880266e-09 -3454.75271945471 -24111.946705421;-1.1e-05 2.49182272265674e-09 -3445.6624844153 -24113.247403059;-1e-05 2.49159397236724e-09 -3436.57175967041 -24114.5446736669;-9e-06 2.49136486796667e-09 -3427.48054651203 -24115.8385170602;-8e-06 2.49113540948759e-09 -3418.38884623222 -24117.1289330549;-7e-06 2.49090559696261e-09 -3409.29666012313 -24118.4159214678;-6e-06 2.49067543042439e-09 -3400.20398947694 -24119.699482116;-5e-06 2.49044490990565e-09 -3391.11083558594 -24120.9796148169;-4e-06 2.49021403543915e-09 -3382.01719974246 -24122.2563193887;-3e-06 2.48998280705769e-09 -3372.92308323891 -24123.5295956499;-2e-06 2.48975122479415e-09 -3363.82848736777 -24124.7994434195;-1e-06 2.48951928868143e-09 -3354.73341342159 -24126.0658625171]  x3=[-2.1e-05 3.74254700615526e-12 -11.156979296135 -79.1361755515133;-2e-05 3.74512559804933e-12 -11.1271448686844 -79.1403760100091;-1.9e-05 3.74770365767753e-12 -11.0973088598183 -79.1445652208925;-1.8e-05 3.75028118467347e-12 -11.0674712737772 -79.1487431835682;-1.7e-05 3.7528581786708e-12 -11.0376321148016 -79.1529098974423;-1.6e-05 3.7554346393033e-12 -11.0077913871323 -79.1570653619226;-1.5e-05 3.75801056620478e-12 -10.9779490950103 -79.1612095764186;-1.4e-05 3.76058595900915e-12 -10.948105242677 -79.1653425403413;-1.3e-05 3.76316081735039e-12 -10.9182598343737 -79.1694642531034;-1.2e-05 3.76573514086255e-12 -10.8884128743422 -79.1735747141189;-1.1e-05 3.76830892917976e-12 -10.8585643668244 -79.1776739228038;-1e-05 3.77088218193624e-12 -10.8287143160625 -79.1817618785754;-9e-06 3.77345489876626e-12 -10.7988627262987 -79.1858385808527;-8e-06 3.77602707930419e-12 -10.7690096017758 -79.1899040290564;-7e-06 3.77859872318445e-12 -10.7391549467364 -79.1939582226087;-6e-06 3.78116983004157e-12 -10.7092987654235 -79.1980011609334;-5e-06 3.78374039951013e-12 -10.6794410620805 -79.2020328434558;-4e-06 3.78631043122479e-12 -10.6495818409508 -79.206053269603;-3e-06 3.7888799248203e-12 -10.6197211062779 -79.2100624388037;-2e-06 3.79144887993148e-12 -10.5898588623059 -79.214060350488;-1e-06 3.79401729619321e-12 -10.5599951132787 -79.2180470040876]  x4=[-2.1e-05 3.0197126057934e-12 -12.5606324026064 -78.9000787577136;-2e-05 3.01615981572906e-12 -12.5308868818028 -78.9048083977287;-1.9e-05 3.01260659700115e-12 -12.5011395800808 -78.9095268236108;-1.8e-05 3.00905295011465e-12 -12.471390501668 -78.9142340346893;-1.7e-05 3.00549887557462e-12 -12.4416396507925 -78.9189300302953;-1.6e-05 3.00194437388618e-12 -12.4118870316825 -78.9236148097612;-1.5e-05 2.99838944555449e-12 -12.3821326485665 -78.9282883724214;-1.4e-05 2.99483409108479e-12 -12.3523765056734 -78.9329507176116;-1.3e-05 2.99127831098237e-12 -12.3226186072321 -78.9376018446691;-1.2e-05 2.9877221057526e-12 -12.2928589574719 -78.942241752933;-1.1e-05 2.98416547590088e-12 -12.2630975606222 -78.9468704417437;-1e-05 2.9806084219327e-12 -12.2333344209129 -78.9514879104435;-9e-06 2.97705094435359e-12 -12.203569542574 -78.9560941583762;-8e-06 2.97349304366915e-12 -12.1738029298357 -78.960689184887;-7e-06 2.96993472038503e-12 -12.1440345869285 -78.9652729893229;-6e-06 2.96637597500696e-12 -12.1142645180831 -78.9698455710325;-5e-06 2.9628168080407e-12 -12.0844927275306 -78.9744069293658;-4e-06 2.95925721999209e-12 -12.0547192195021 -78.9789570636747;-3e-06 2.95569721136705e-12 -12.0249439982292 -78.9834959733124;-2e-06 2.9521367826715e-12 -11.9951670679436 -78.9880236576339;-1e-06 2.94857593441149e-12 -11.9653884328773 -78.9925401159956]  x5=2.03919101606495e-05  V1=[0 0 0 2.827e-09 2.436e+04 2.436e+04;0 0 0 377 377 377;1.571 1.571 1.571 -0.5179 -0.1443 -1.715]  V2=[0 0 0 2.868e-09 2.436e+04 2.436e+04;0 0 0 377 377 377;1.571 1.571 1.571 -0.5251 -0.1443 -1.715]  I1=[0 0 0 7.018e-12 79.92 79.92;0 0 0 377 377 377;1.571 1.571 1.571 -1.622 -0.1386 -1.709]  I2=[0 0 0 7.946e-12 79.89 79.89;0 0 0 377 377 377;1.571 1.571 1.571 0.3547 -0.1565 -1.727]  nHarmo=2  Measurements=None  Decoupling=off  VsMag0=0  VrMag0=0  VsAngle0=0  VrAngle0=0  IsMag0=0  IrMag0=0  IsAngle0=0  IrAngle0=0
  Ground3 : spsGroundLib/Ground  LConnTagsString=a
  "Grounding Transformer " : spsGroundingTransformerLib/Grounding Transformer   UNITS=pu  NominalPower="[100e6   60]"  NominalVoltage=25e3  ZeroSequenceImpedance_pu=[0.025 0.75]  MagnetizationBranch_pu=[500 500]  ZeroSequenceImpedance_SI=[0.052083 589.05]  MagnetizationBranch_SI=[1041.7 3.927e+005]  Measurements=None
  A : PMIOPort  Side=Left
  B : PMIOPort  Port=2  Side=Left
  C : PMIOPort  Port=3  Side=Left
  connections:
  "3.3ohms "/RConn1 -- Ground3/LConn1
  120 kV / 25 kV 47 MVA/LConn1 -- 120kV 2500MVA/RConn1
  120 kV / 25 kV 47 MVA/LConn2 -- 120kV 2500MVA/RConn2
  120 kV / 25 kV 47 MVA/LConn3 -- 120kV 2500MVA/RConn3
  120 kV / 25 kV 47 MVA/RConn1 -- "Grounding Transformer "/LConn1 -- 14-km Feeder/RConn1 -- 30-MW 2-Mvar Load/LConn1
  120 kV / 25 kV 47 MVA/RConn2 -- "Grounding Transformer "/LConn2 -- 14-km Feeder/RConn2 -- 30-MW 2-Mvar Load/LConn2
  120 kV / 25 kV 47 MVA/RConn3 -- "Grounding Transformer "/LConn3 -- 14-km Feeder/RConn3 -- 30-MW 2-Mvar Load/LConn3
  5-km Feeder/RConn1 -- 14-km Feeder/LConn1 -- 2-MW Load/LConn1
  5-km Feeder/RConn2 -- 14-km Feeder/LConn2 -- 2-MW Load/LConn2
  5-km Feeder/RConn3 -- 14-km Feeder/LConn3 -- 2-MW Load/LConn3
  A/RConn1 -- 5-km Feeder/LConn1
  B/RConn1 -- 5-km Feeder/LConn2
  C/RConn1 -- 5-km Feeder/LConn3
  "Grounding Transformer "/RConn1 -- "3.3ohms "/LConn1

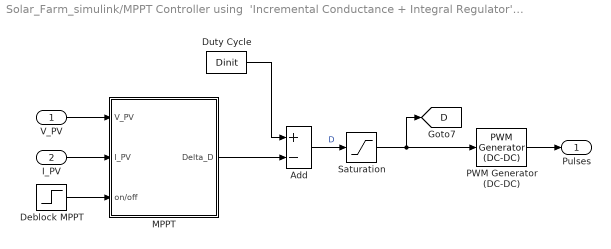
== system Solar_Farm_simulink/MPPT Controller using  'Incremental Conductance + Integral Regulator'  technique  ==
  V_PV : Inport
  I_PV : Inport  Port=2
  Add : Sum  Inputs=+-
  Deblock MPPT : Step  Time=0.4  SampleTime=0
  Duty Cycle : Constant  Value=Dinit
  MPPT : Subsystem
  PWM Generator (DC-DC) : spsPWMGeneratorDCDCLib/PWM Generator (DC-DC)  Fsw=fc  Ts=Ts_Power
  Saturation : Saturate  UpperLimit=1  LowerLimit=0
  Pulses : Outport  VectorParamsAs1DForOutWhenUnconnected=off
  tag scope: D=global
  wires:
  V_PV/1 -> MPPT/1(V_PV)
  I_PV/1 -> MPPT/2(I_PV)
  PWM Generator (DC-DC)/1 -> Pulses/1
  Deblock MPPT/1 -> MPPT/3(on/off)
  Saturation/1 -> PWM Generator (DC-DC)/1, [D]
  Add/1 -> Saturation/1  "D"
  MPPT/1(Delta_D) -> Add/2
  Duty Cycle/1 -> Add/1

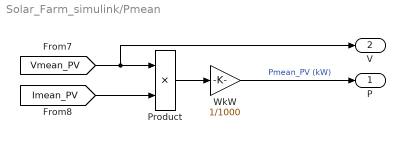
== system Solar_Farm_simulink/Pmean ==
  Product : Product  RndMeth=Zero
  WkW : Gain  Gain=1/1000
  P : Outport  VectorParamsAs1DForOutWhenUnconnected=off
  V : Outport  Port=2  VectorParamsAs1DForOutWhenUnconnected=off
  wires:
  [Vmean_PV] -> Product/1, V/1
  Product/1 -> WkW/1
  [Imean_PV] -> Product/2
  WkW/1 -> P/1  "Pmean_PV (kW)"

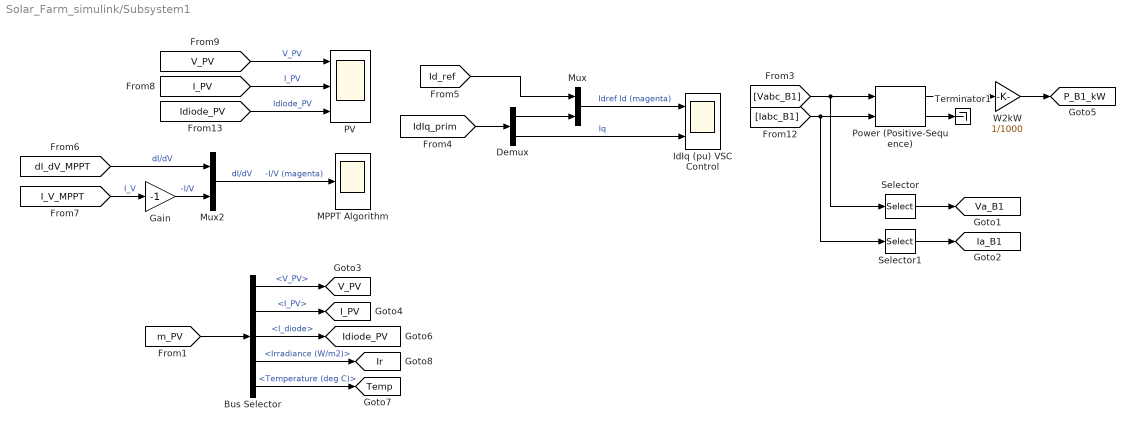
== system Solar_Farm_simulink/Subsystem1 ==
  Bus Selector : BusSelector  OutputSignals=V_PV,I_PV,I_diode,Irradiance (W/m2),Temperature (deg C)
  Demux : Demux  Outputs=2
  Gain : Gain  Gain=-1
  IdIq (pu) VSC Control : Scope  NumInputPorts=2
  MPPT Algorithm : Scope
  Mux : Mux  Inputs=2
  Mux2 : Mux  Inputs=2
  PV : Scope  NumInputPorts=3
  Power (Positive-Sequence) : spsPowerPositiveSequenceLib/Power (Positive-Sequence)  Freq=60  Vinit=[0, 0]  Iinit=[0, 0]  Ts=Ts_Control
  Selector : Selector  InputPortWidth=3  IndexOptions=Index vector (dialog)  Indices=[1]  OutputSizes=1
  Selector1 : Selector  InputPortWidth=3  IndexOptions=Index vector (dialog)  Indices=[1]  OutputSizes=1
  Terminator1 : Terminator
  W2kW : Gain  Gain=1/1000
  tag scope: I_PV=global, Ia_B1=global, Idiode_PV=global, Ir=global, P_B1_kW=global, Temp=global, V_PV=global, Va_B1=global
  wires:
  [Vabc_B1] -> Power (Positive-Sequence)/1, Selector/1
  [Iabc_B1] -> Power (Positive-Sequence)/2, Selector1/1
  Power (Positive-Sequence)/1 -> W2kW/1
  [I_V_MPPT] -> Gain/1  "I_V"
  [IdIq_prim] -> Demux/1
  [Id_ref] -> Mux/1
  Demux/1 -> Mux/2
  Mux/1 -> IdIq (pu) VSC Control/1  "Idref Id (magenta)"
  Demux/2 -> IdIq (pu) VSC Control/2  "Iq"
  Selector/1 -> [Va_B1]
  Selector1/1 -> [Ia_B1]
  [V_PV] -> PV/1  "V_PV"
  [I_PV] -> PV/2  "I_PV"
  [Idiode_PV] -> PV/3  "Idiode_PV"
  [dI_dV_MPPT] -> Mux2/1  "dI/dV"
  Gain/1 -> Mux2/2  "-I/V"
  Mux2/1 -> MPPT Algorithm/1  "dI/dV     -I/V (magenta)"
  W2kW/1 -> [P_B1_kW]
  [m_PV] -> Bus Selector/1
  Bus Selector/1 -> [V_PV]  "<V_PV>"
  Bus Selector/2 -> [I_PV]  "<I_PV>"
  Bus Selector/4 -> [Ir]  "<Irradiance (W/m2)>"
  Bus Selector/3 -> [Idiode_PV]  "<I_diode>"
  Bus Selector/5 -> [Temp]  "<Temperature (deg C)>"
  Power (Positive-Sequence)/2 -> Terminator1/1

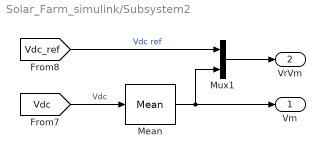
== system Solar_Farm_simulink/Subsystem2 ==
  Mean : spsMeanLib/Mean  Freq=60  Vinit=0  Ts=Ts_Control
  Mux1 : Mux  Inputs=2
  Vm : Outport  VectorParamsAs1DForOutWhenUnconnected=off
  VrVm : Outport  Port=2  VectorParamsAs1DForOutWhenUnconnected=off
  wires:
  [Vdc_ref] -> Mux1/1  "Vdc ref"
  [Vdc] -> Mean/1  "Vdc"
  Mux1/1 -> VrVm/1
  Mean/1 -> Mux1/2, Vm/1

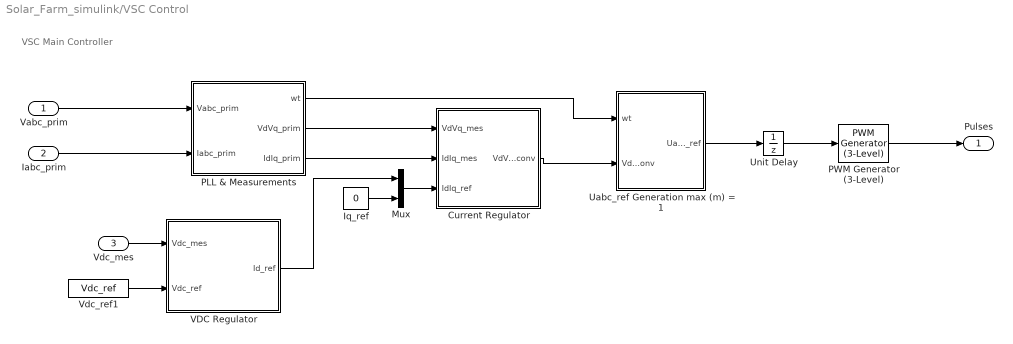
== system Solar_Farm_simulink/VSC Control ==
  note: VSC Main Controller
  Vabc_prim : Inport  PortDimensions=3
  Iabc_prim : Inport  Port=2  PortDimensions=3
  Vdc_mes : Inport  Port=3  PortDimensions=1
  Current Regulator : Subsystem
  Iq_ref : Constant  Value=0
  Mux : Mux  Inputs=2
  PLL & Measurements : Subsystem
  PWM Generator (3-Level) : spsPWMGenerator3LevelLib/PWM Generator (3-Level)  ModulatorType=Three-phase bridge (12 pulses)  ModulatorMode=Unsynchronized  nF=27  Fc=33*60  ModulatingSignals=off  m=0.8  Freq=60  Phase=0  Ts=Ts_Power
  Uabc_ref Generation max (m) = 1 : Subsystem
  Unit Delay : UnitDelay  SampleTime=Ts_Control  HasFrameUpgradeWarning=on
  VDC Regulator : Subsystem
  Vdc_ref1 : Constant  Value=Vdc_ref
  Pulses : Outport  VectorParamsAs1DForOutWhenUnconnected=off
  wires:
  VDC Regulator/1(Id_ref) -> Mux/1
  PLL & Measurements/1(wt) -> Uabc_ref Generation max (m) = 1/1(wt)
  Current Regulator/1(VdVq_conv) -> Uabc_ref Generation max (m) = 1/2(VdVq_conv)
  Iq_ref/1 -> Mux/2
  Mux/1 -> Current Regulator/3(IdIq_ref)
  PLL & Measurements/3(IdIq_prim) -> Current Regulator/2(IdIq_mes)
  PLL & Measurements/2(VdVq_prim) -> Current Regulator/1(VdVq_mes)
  Vdc_mes/1 -> VDC Regulator/1(Vdc_mes)
  Vabc_prim/1 -> PLL & Measurements/1(Vabc_prim)
  Iabc_prim/1 -> PLL & Measurements/2(Iabc_prim)
  Unit Delay/1 -> PWM Generator (3-Level)/1
  PWM Generator (3-Level)/1 -> Pulses/1
  Uabc_ref Generation max (m) = 1/1(Uabc_ref) -> Unit Delay/1
  Vdc_ref1/1 -> VDC Regulator/2(Vdc_ref)

== system Solar_Farm_simulink/info ==

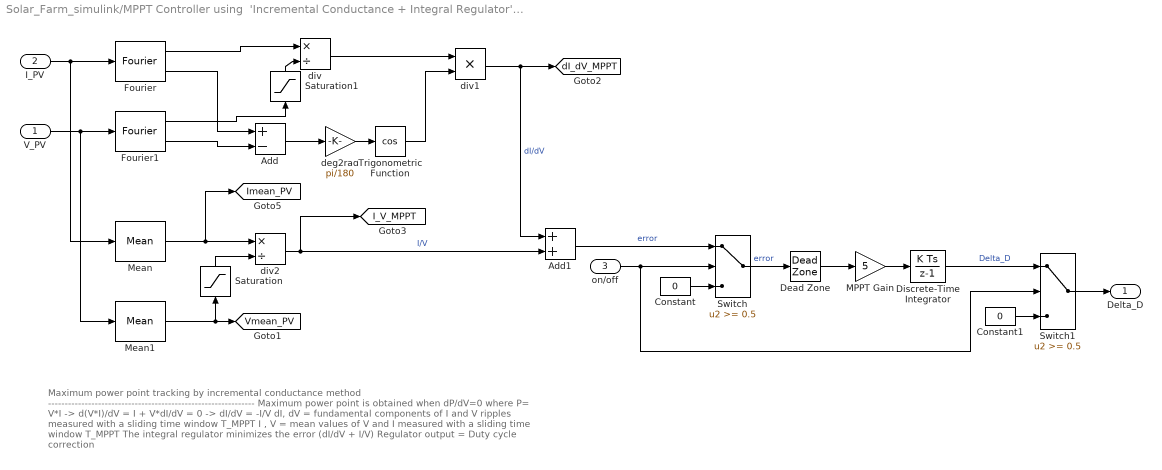
== system Solar_Farm_simulink/MPPT Controller using  'Incremental Conductance + Integral Regulator'  technique /MPPT ==
  note: Maximum power point tracking by incremental conductance method
      | --------------------------------------------------------------
      | Maximum power point is obtained when dP/dV=0  where P= V*I
      | -> d(V*I)/dV = I + V*dI/dV = 0
      | -> dI/dV = -I/V
      |
      | dI, dV  = fundamental components of I and V ripples measured with a sliding time window T_MPPT
      | I , V   = mean values of V and I measured with a sliding time window T_MPPT
      |
      | The integral regulator minimizes the error (dI/dV + I/V)
      | Regulator output = Duty cycle correction
  V_PV : Inport
  I_PV : Inport  Port=2
  on/off : Inport  Port=3
  Add : Sum  Inputs=+-
  Add1 : Sum
  Constant : Constant  Value=0
  Constant1 : Constant  Value=0
  Dead Zone : DeadZone  LowerValue=-0.05  UpperValue=0.05
  Discrete-Time Integrator : DiscreteIntegrator  SampleTime=Ts_Control  LimitOutput=on  UpperSaturationLimit=1  LowerSaturationLimit=-1  ICPrevOutput=DiscIntNeverNeededParam  ICPrevScaledInput=DiscIntNeverNeededParam
  Fourier : spsFourierLib/Fourier  Freq=1/T_MPPT  n=1  InInit=[0, 0]  Ts=Ts_Control
  Fourier1 : spsFourierLib/Fourier  Freq=1/T_MPPT  n=1  InInit=[0, 0]  Ts=Ts_Control
  MPPT Gain : Gain  Gain=5
  Mean : spsMeanLib/Mean  Freq=1/T_MPPT  Vinit=0  Ts=Ts_Control
  Mean1 : spsMeanLib/Mean  Freq=1/T_MPPT  Vinit=0  Ts=Ts_Control
  Saturation : Saturate  UpperLimit=inf  LowerLimit=eps
  Saturation1 : Saturate  UpperLimit=inf  LowerLimit=eps
  Switch : Switch  Threshold=0.5  SaturateOnIntegerOverflow=off  InputSameDT=off
  Switch1 : Switch  Threshold=0.5  SaturateOnIntegerOverflow=off  InputSameDT=off
  Trigonometric Function : Trigonometry  Operator=cos
  deg2rad : Gain  Gain=pi/180
  div : Product  Inputs=*/  RndMeth=Zero
  div1 : Product  Inputs=**  RndMeth=Zero
  div2 : Product  Inputs=*/  RndMeth=Zero
  Delta_D : Outport  VectorParamsAs1DForOutWhenUnconnected=off
  tag scope: I_V_MPPT=global, Imean_PV=global, Vmean_PV=global, dI_dV_MPPT=global
  wires:
  Dead Zone/1 -> MPPT Gain/1
  Switch/1 -> Dead Zone/1  "error"
  Saturation1/1 -> div/2
  Saturation/1 -> div2/2
  Switch1/1 -> Delta_D/1
  on/off/1 -> Switch/2, Switch1/2
  Constant1/1 -> Switch1/3
  Discrete-Time Integrator/1 -> Switch1/1  "Delta_D"
  Constant/1 -> Switch/3
  MPPT Gain/1 -> Discrete-Time Integrator/1
  Add1/1 -> Switch/1  "error"
  div2/1 -> Add1/2, [I_V_MPPT]  "I/V"
  Mean1/1 -> Saturation/1, [Vmean_PV]
  Mean/1 -> div2/1, [Imean_PV]
  div1/1 -> Add1/1, [dI_dV_MPPT]  "dI/dV"
  Trigonometric Function/1 -> div1/2
  div/1 -> div1/1
  deg2rad/1 -> Trigonometric Function/1
  Add/1 -> deg2rad/1
  Fourier1/1 -> Saturation1/1
  Fourier1/2 -> Add/2
  Fourier/2 -> Add/1
  V_PV/1 -> Mean1/1, Fourier1/1
  I_PV/1 -> Mean/1, Fourier/1
  Fourier/1 -> div/1
